simulink model "Complete_DAC_mod3_CRFF_CTExample"  (Simulink 7.9)
settings: Solver=ode45  StartTime=0.0  StopTime=simu.trantime  RelTol=1e-3
values from neighbouring files (symbols this model uses):
  dc = 0    [CRFF_CTExample.m]
  Fs = fb*2*OSR    (= 3072000)    [CRFF_CTExample.m]
  OSR = 64    [CRFF_CTExample.m]    (also in MakeModulator_CTExample.m)
  sinamp = 1/sqrt(2)    [CRFF_CTExample.m]
  sinfreq = 12e3    (= 12000)    [CRFF_CTExample.m]
undefined symbols (not defined in the file or in its folder): a, b, c, dac, g, mod
libraries: simulink x9, dspsigops x6, dsparch4 x1, dspmtrx3 x1, commnoisgen2 x1, dspsrcs4 x1
settings Model: Creator=amyles  LastModifiedBy=Arnaldi Isacco
settings SolverCC: ZeroCrossAlgorithm=Adaptive  AutoInsertRateTranBlk=on
settings DataIOCC: MaxDataPoints=50000  SaveOutput=off  SaveTime=off
settings OptimizationCC: InlineParams=on
settings DebuggingCC: UnderspecifiedInitializationDetection=Simplified  InvalidFcnCallConnMsg=none  StrictBusMsg=ErrorOnBusTreatedAsVector
settings ModelReferenceCC: ModelReferenceNumInstancesAllowed=Single
settings CodeAppCC: CustomSymbolStrType=$N$R$M_T
settings GRTTargetCC: CombineOutputUpdateFcns=off  GRTInterface=on

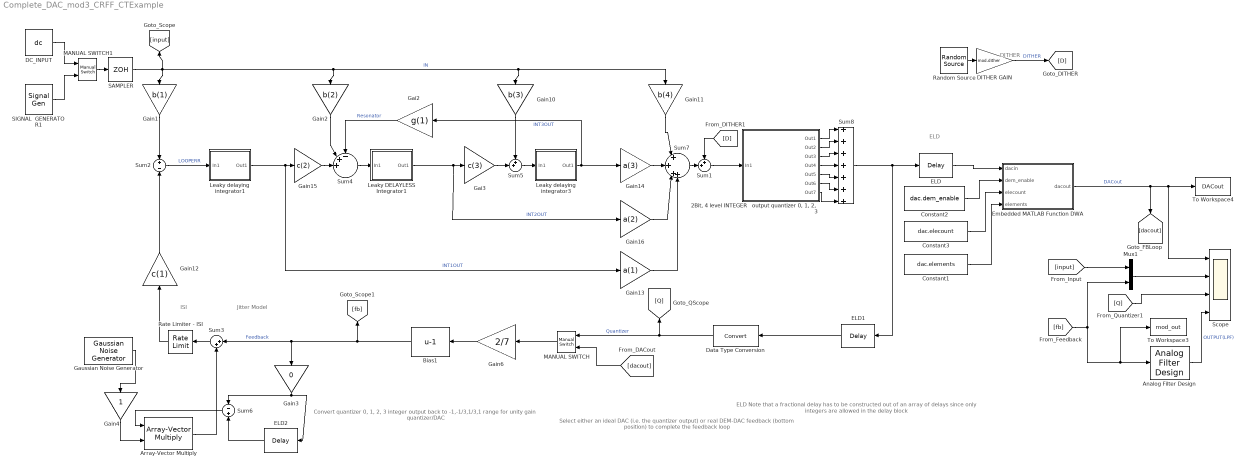
== system Complete_DAC_mod3_CRFF_CTExample ==
  note: DITHER
  note: Convert quantizer 0, 1, 2, 3 integer
      | output back  to -1,-1/3,1/3,1 range for
      | unity gain quantizer/DAC
  note: Select either an ideal DAC
      | (i.e. the quantizer output) or real
      | DEM-DAC feedback (bottom position) to
      | complete the feedback loop
  note: ELD
      | Note that a fractional
      | delay has to be
      | constructed out of
      | an array of delays
      | since only integers
      | are allowed in the
      | delay block
  note: ELD
  note: Jitter Model
  note: ISI
  "2Bit, 4 level INTEGER   output quantizer 0, 1, 2, 3" : Subsystem
  Analog Filter Design : dsparch4/Analog Filter Design  method=Butterworth  filttype=Lowpass  N=8  Wlo=pi*(Fs/OSR)  Whi=80  Rp=2  Rs=40
      settings: AttributesFormatString=Low-pass filter the loop output\nto illustrate intuitively how the\npulse density modulated +1/-1\noutput stream does indeed capture\nthe input signal
  Array-Vector Multiply : dspmtrx3/Array-Vector Multiply  mode=Mute  saveAsFlag=0  Dimension=2  V_Source=Input port  V_VectFromMask=[0.5 0.25]  firstCoeffSignedness=Auto  firstCoeffDataTypeStr=Inherit: Same word length as input  firstCoeffLastDataTypeStr=Inherit: Same word length as input  firstCoeffMin=[]  firstCoeffMax=[]  outputSignedness=Auto  outputDataTypeStr=Inherit: Same as product output  outputLastDataTypeStr=Inherit: Same as product output  outputMin=[]  outputMax=[]  accumSignedness=Auto  prodOutputSignedness=Auto  roundingMode=Floor  overflowMode=off
  Bias1 : Bias  Bias=-1
  Constant1 : Constant  Value=dac.elements  SampleTime=1/Fs
  Constant2 : Constant  Value=dac.dem_enable  SampleTime=1/Fs
  Constant3 : Constant  Value=dac.elecount  SampleTime=1/Fs
  DC_INPUT : Constant  Value=dc  VectorParams1D=off  OutDataTypeStr=double  SampleTime=1/Fs
  DITHER GAIN : Gain  Gain=mod.dither  SampleTime=1/Fs
  Data Type Conversion : DataTypeConversion  SampleTime=1/Fs  LockScale=on
  ELD : dspsigops/Delay  InputProcessing=Inherited (this choice will be removed - see release notes)  dly_unit=Samples  delay=0  ic_detail=off  dif_ic_for_ch=off  dif_ic_for_dly=off  ic=0  reset_popup=None
  ELD1 : dspsigops/Delay  InputProcessing=Inherited (this choice will be removed - see release notes)  dly_unit=Samples  delay=0  ic_detail=off  dif_ic_for_ch=off  dif_ic_for_dly=off  ic=0  reset_popup=None
  ELD2 : dspsigops/Delay  InputProcessing=Inherited (this choice will be removed - see release notes)  dly_unit=Samples  delay=1  ic_detail=off  dif_ic_for_ch=off  dif_ic_for_dly=off  ic=0  reset_popup=None
  Embedded MATLAB Function DWA : MATLAB Function  TreatAsAtomicUnit=on
  Gai2 : Gain  Gain=g(1)
  Gai3 : Gain  Gain=c(3)
  Gain1 : Gain  Gain=b(1)  SampleTime=1/Fs
  Gain10 : Gain  Gain=b(3)  SampleTime=1/Fs
  Gain11 : Gain  Gain=b(4)  SampleTime=1/Fs
  Gain12 : Gain  Gain=c(1)  SampleTime=1/Fs
  Gain13 : Gain  Gain=a(1)
  Gain14 : Gain  Gain=a(3)
  Gain15 : Gain  Gain=c(2)
  Gain16 : Gain  Gain=a(2)
  Gain2 : Gain  Gain=b(2)  SampleTime=1/Fs
  Gain3 : Gain  Gain=0  SampleTime=1/Fs
  Gain4 : Gain  SampleTime=1/Fs
  Gain6 : Gain  Gain=2/7  SampleTime=1/Fs
  Gaussian Noise Generator : commnoisgen2/Gaussian Noise Generator  m=50e-12  d=50  s=40  Ts=1/Fs  frameBased=off  sampPerFrame=1  orient=on  outDataType=double
  Leaky DELAYLESS Integrator1 : Subsystem
  Leaky delaying integrator1 : Subsystem
  Leaky delaying integrator3 : Subsystem
  MANUAL SWITCH : simulink/Signal Routing/Manual Switch  sw=0  action=0  varsize=off
      settings: AttributesFormatString=Double click to\nselect the desired\ninput
  MANUAL SWITCH1 : simulink/Signal Routing/Manual Switch  sw=0  action=0  varsize=off
      settings: AttributesFormatString=Double click to\nselect the desired\ninput
  Mux1 : Mux  Inputs=2
  Random Source : dspsrcs4/Random Source  SrcType=Uniform  NormMethod=Ziggurat  CltLength=12  MinVal=-1  MaxVal=1  MeanVal=0  VarVal=1  RepMode=Not repeatable  rawSeed=1  IsInherit=off  SampMode=Discrete  SampTime=1/Fs  SampFrame=1  DataType=Double  OutComplex=Real
  Rate Limiter - ISI : RateLimiter  RisingSlewLimit=inf  FallingSlewLimit=-inf  SampleTimeMode=inherited
  SAMPLER : ZeroOrderHold  SampleTime=1/Fs
  SIGNAL  GENERATOR1 : SignalGenerator  Amplitude=sinamp  Frequency=sinfreq  VectorParams1D=off
  Scope : Scope  NumInputPorts=4
      settings: YMin=0~-1~-1~-1  YMax=3.5~1~1~1
  Sum1 : Sum  Inputs=++|  SampleTime=1/Fs
  Sum2 : Sum  Inputs=+-  SampleTime=1/Fs
  Sum3 : Sum  Inputs=|++  SampleTime=1/Fs
  Sum4 : Sum  Inputs=-++||
  Sum5 : Sum  Inputs=++|
  Sum6 : Sum  Inputs=-+  SampleTime=1/Fs
  Sum7 : Sum  Inputs=|+|+|++
  Sum8 : Sum  Inputs=+++++++  SampleTime=1/Fs
  To Workspace3 : ToWorkspace  VariableName=mod_out  SampleTime=-1
  To Workspace4 : ToWorkspace  VariableName=DACout  SampleTime=-1
  wires:
  Random Source/1 -> DITHER GAIN/1
  DITHER GAIN/1 -> [D]  "DITHER"
  MANUAL SWITCH/1 -> Gain6/1
  Gain6/1 -> Bias1/1
  [dacout] -> MANUAL SWITCH/2
  Embedded MATLAB Function DWA/1(dacout) -> [dacout], To Workspace4/1, Scope/1  "DACout"
  [input] -> Mux1/1
  [fb] -> Mux1/2, Analog Filter Design/1, To Workspace3/1
  Mux1/1 -> Scope/2
  [Q] -> Scope/3
  Analog Filter Design/1 -> Scope/4  "OUTPUT(LPF)"
  Constant2/1 -> Embedded MATLAB Function DWA/2(dem_enable)
  Constant3/1 -> Embedded MATLAB Function DWA/3(elecount)
  Constant1/1 -> Embedded MATLAB Function DWA/4(elements)
  SAMPLER/1 -> Gain11/1, Gain10/1, Gain2/1, Gain1/1, [input]  "IN"
  Gain15/1 -> Sum4/3
  Leaky DELAYLESS Integrator1/1(Out1) -> Gai3/1, Gain16/1  "INT2OUT"
  Gai3/1 -> Sum5/2
  Leaky delaying integrator3/1(Out1) -> Gain14/1, Gai2/1  "INT3OUT"
  Gain12/1 -> Sum2/2
  Gain1/1 -> Sum2/1
  Gain2/1 -> Sum4/2
  Gai2/1 -> Sum4/1  "Resonator"
  Gain10/1 -> Sum5/1
  Sum2/1 -> Leaky delaying integrator1/1(In1)  "LOOPERR"
  Sum5/1 -> Leaky delaying integrator3/1(In1)
  Sum4/1 -> Leaky DELAYLESS Integrator1/1(In1)
  Leaky delaying integrator1/1(Out1) -> Gain15/1, Gain13/1  "INT1OUT"
  Gain14/1 -> Sum7/2
  Gain11/1 -> Sum7/1
  Gain16/1 -> Sum7/3
  Gain13/1 -> Sum7/4
  Sum7/1 -> Sum1/2
  Sum1/1 -> "2Bit, 4 level INTEGER   output quantizer 0, 1, 2, 3"/1(In1)
  [D] -> Sum1/1
  Data Type Conversion/1 -> MANUAL SWITCH/1, [Q]  "Quantizer"
  Bias1/1 -> [fb], Sum3/1, Gain3/1  "Feedback"
  Sum8/1 -> ELD/1, ELD1/1
  "2Bit, 4 level INTEGER   output quantizer 0, 1, 2, 3"/1(Out1) -> Sum8/1
  "2Bit, 4 level INTEGER   output quantizer 0, 1, 2, 3"/2(Out2) -> Sum8/2
  "2Bit, 4 level INTEGER   output quantizer 0, 1, 2, 3"/3(Out3) -> Sum8/3
  "2Bit, 4 level INTEGER   output quantizer 0, 1, 2, 3"/4(Out4) -> Sum8/4
  "2Bit, 4 level INTEGER   output quantizer 0, 1, 2, 3"/5(Out5) -> Sum8/5
  "2Bit, 4 level INTEGER   output quantizer 0, 1, 2, 3"/6(Out6) -> Sum8/6
  "2Bit, 4 level INTEGER   output quantizer 0, 1, 2, 3"/7(Out7) -> Sum8/7
  ELD/1 -> Embedded MATLAB Function DWA/1(dacin)
  Gain3/1 -> Sum6/1, ELD2/1
  ELD2/1 -> Sum6/2
  Sum6/1 -> Array-Vector Multiply/1
  Array-Vector Multiply/1 -> Sum3/2
  Sum3/1 -> Rate Limiter - ISI/1
  Rate Limiter - ISI/1 -> Gain12/1
  Gain4/1 -> Array-Vector Multiply/2
  Gaussian Noise Generator/1 -> Gain4/1
  ELD1/1 -> Data Type Conversion/1
  DC_INPUT/1 -> MANUAL SWITCH1/1
  SIGNAL  GENERATOR1/1 -> MANUAL SWITCH1/2
  MANUAL SWITCH1/1 -> SAMPLER/1

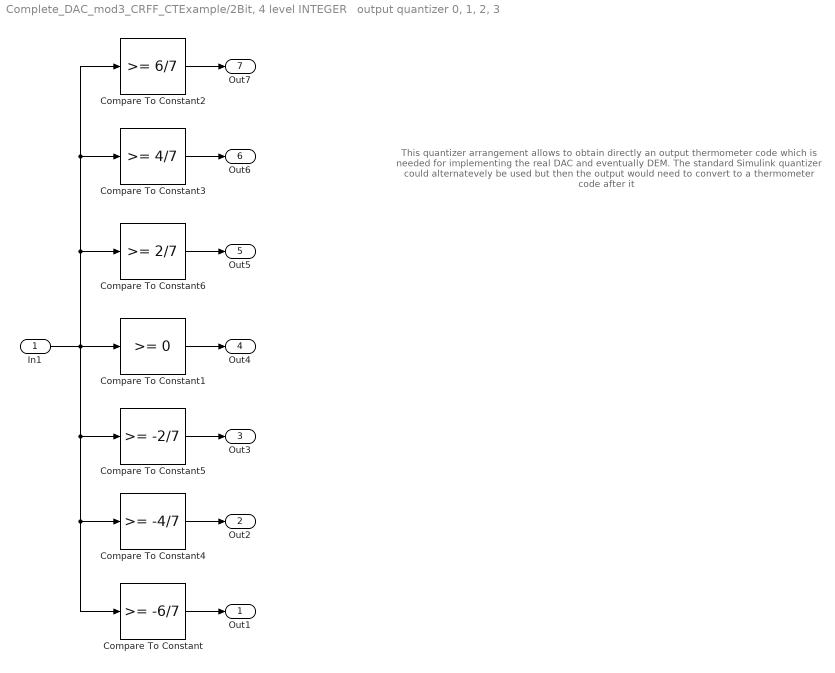
== system Complete_DAC_mod3_CRFF_CTExample/2Bit, 4 level INTEGER   output quantizer 0, 1, 2, 3 ==
  note: This quantizer arrangement allows to obtain directly
      | an output thermometer code which is needed for implementing
      | the real DAC and eventually DEM. The standard Simulink
      | quantizer could alternatevely be used but then the output
      | would need to convert to a thermometer code after it
  In1 : Inport
  Compare To Constant : simulink/Logic and Bit Operations/Compare To Constant  relop=>=  const=-6/7  OutDataTypeStr=uint8
  Compare To Constant1 : simulink/Logic and Bit Operations/Compare To Constant  relop=>=  const=0  OutDataTypeStr=uint8
  Compare To Constant2 : simulink/Logic and Bit Operations/Compare To Constant  relop=>=  const=6/7  OutDataTypeStr=uint8
  Compare To Constant3 : simulink/Logic and Bit Operations/Compare To Constant  relop=>=  const=4/7  OutDataTypeStr=uint8
  Compare To Constant4 : simulink/Logic and Bit Operations/Compare To Constant  relop=>=  const=-4/7  OutDataTypeStr=uint8
  Compare To Constant5 : simulink/Logic and Bit Operations/Compare To Constant  relop=>=  const=-2/7  OutDataTypeStr=uint8
  Compare To Constant6 : simulink/Logic and Bit Operations/Compare To Constant  relop=>=  const=2/7  OutDataTypeStr=uint8
  Out1 : Outport
  Out2 : Outport  Port=2
  Out3 : Outport  Port=3
  Out4 : Outport  Port=4
  Out5 : Outport  Port=5
  Out6 : Outport  Port=6
  Out7 : Outport  Port=7
  wires:
  In1/1 -> Compare To Constant1/1, Compare To Constant2/1, Compare To Constant3/1, Compare To Constant6/1, Compare To Constant5/1, Compare To Constant/1, Compare To Constant4/1
  Compare To Constant2/1 -> Out7/1
  Compare To Constant3/1 -> Out6/1
  Compare To Constant6/1 -> Out5/1
  Compare To Constant1/1 -> Out4/1
  Compare To Constant4/1 -> Out2/1
  Compare To Constant5/1 -> Out3/1
  Compare To Constant/1 -> Out1/1

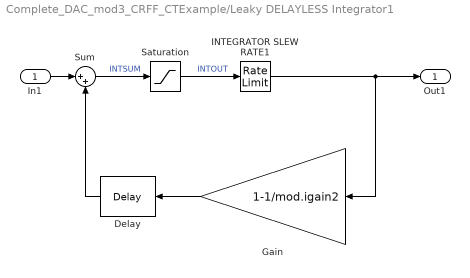
== system Complete_DAC_mod3_CRFF_CTExample/Leaky DELAYLESS Integrator1 ==
  In1 : Inport
  Delay : dspsigops/Delay  InputProcessing=Inherited (this choice will be removed - see release notes)  dly_unit=Samples  delay=1  ic_detail=off  dif_ic_for_ch=off  dif_ic_for_dly=off  ic=0  reset_popup=None
  Gain : Gain  Gain=1-1/mod.igain2
      settings: AttributesFormatString=Integrator leakage
  INTEGRATOR SLEW RATE1 : RateLimiter  RisingSlewLimit=mod.isr2  FallingSlewLimit=-(mod.isr2)  SampleTimeMode=inherited
  Saturation : Saturate  UpperLimit=mod.isat2  LowerLimit=-(mod.isat2)
  Sum : Sum  Inputs=|++  SampleTime=1/Fs
      settings: AttributesFormatString=Integrator summer
  Out1 : Outport
  wires:
  In1/1 -> Sum/1
  Gain/1 -> Delay/1
  Sum/1 -> Saturation/1  "INTSUM"
  Delay/1 -> Sum/2
  Saturation/1 -> INTEGRATOR SLEW RATE1/1  "INTOUT"
  INTEGRATOR SLEW RATE1/1 -> Gain/1, Out1/1

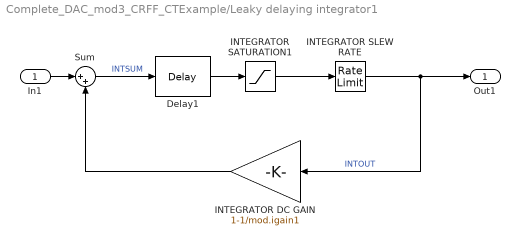
== system Complete_DAC_mod3_CRFF_CTExample/Leaky delaying integrator1 ==
  In1 : Inport
  Delay1 : dspsigops/Delay  InputProcessing=Inherited (this choice will be removed - see release notes)  dly_unit=Samples  delay=1  ic_detail=off  dif_ic_for_ch=off  dif_ic_for_dly=off  ic=0  reset_popup=None
  INTEGRATOR SATURATION1 : Saturate  UpperLimit=mod.isat1  LowerLimit=-(mod.isat1)
  INTEGRATOR SLEW RATE : RateLimiter  RisingSlewLimit=mod.isr1  FallingSlewLimit=-(mod.isr1)  SampleTimeMode=inherited
  INTEGRATOR DC GAIN : Gain  Gain=1-1/mod.igain1  SampleTime=1/Fs
      settings: AttributesFormatString=Integrator leakage\n(model finite integrator dc/LF\ngain in analog modulators)
  Sum : Sum  Inputs=|++  SampleTime=1/Fs
      settings: AttributesFormatString=Integrator summer
  Out1 : Outport
  wires:
  Sum/1 -> Delay1/1  "INTSUM"
  INTEGRATOR DC GAIN/1 -> Sum/2
  INTEGRATOR SATURATION1/1 -> INTEGRATOR SLEW RATE/1
  In1/1 -> Sum/1
  Delay1/1 -> INTEGRATOR SATURATION1/1
  INTEGRATOR SLEW RATE/1 -> Out1/1, INTEGRATOR DC GAIN/1  "INTOUT"

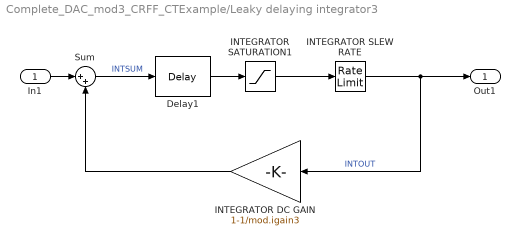
== system Complete_DAC_mod3_CRFF_CTExample/Leaky delaying integrator3 ==
  In1 : Inport
  Delay1 : dspsigops/Delay  InputProcessing=Inherited (this choice will be removed - see release notes)  dly_unit=Samples  delay=1  ic_detail=off  dif_ic_for_ch=off  dif_ic_for_dly=off  ic=0  reset_popup=None
  INTEGRATOR SATURATION1 : Saturate  UpperLimit=mod.isat3  LowerLimit=-(mod.isat3)
  INTEGRATOR SLEW RATE : RateLimiter  RisingSlewLimit=mod.isr3  FallingSlewLimit=-(mod.isr3)  SampleTimeMode=inherited
  INTEGRATOR DC GAIN : Gain  Gain=1-1/mod.igain3
      settings: AttributesFormatString=Integrator leakage\n(model finite integrator dc/LF\ngain in analog modulators)
  Sum : Sum  Inputs=|++  SampleTime=1/Fs
      settings: AttributesFormatString=Integrator summer
  Out1 : Outport
  wires:
  Sum/1 -> Delay1/1  "INTSUM"
  INTEGRATOR DC GAIN/1 -> Sum/2
  INTEGRATOR SATURATION1/1 -> INTEGRATOR SLEW RATE/1
  In1/1 -> Sum/1
  Delay1/1 -> INTEGRATOR SATURATION1/1
  INTEGRATOR SLEW RATE/1 -> Out1/1, INTEGRATOR DC GAIN/1  "INTOUT"

== matlab function Embedded MATLAB Function DWA ==
  data: dacin input double; dacout output double; dem_enable input double; elecount input double; elements input double
function dacout = DAC(dacin, dem_enable, elecount, elements)
%% ------------------- DATA WEIGHTING AVERAGING DEM -----------------------
%
% This function performs DWA DEM and assumes the routines load_par has been
% compiled in order to load the dac structure needed for the code to function.

%% FUNCTION CODE:

persistent dwa_pointer; % Persistent rotator state

% DEM DISABLED:

if isempty(dwa_pointer) || (dem_enable == 0)
    dwa_pointer = 1;    % Reset if not rotating
end

% DEM ENABLED:

dacout = 0.0;

for indx = 1:1:dacin
    dacout = dacout + elements(dwa_pointer);
    dwa_pointer = dwa_pointer + 1;
    if (dwa_pointer > elecount)
        dwa_pointer = 1;
    end
end

end
